simulink model "Alpha3"  (R2024a)
settings: Solver=FixedStepDiscrete  StartTime=0.0  StopTime=44100  RelTol=1e-3
PreLoadFcn:
  | t = linspace(0,256,4096)';
model workspace (MAT data in the model file):
  filter_nr_interpolations = Simulink.Parameter
  filter_nr_interpolations.Value = 4
  filter_nr_interpolations.Complexity = 'real'
  filter_nr_interpolations.Dimensions = [1 1]
  filter_nr_interpolations.Description = 'Number of interpolations applied by the low-pass filter'
  filter_nr_interpolations.DataType = 'uint8'
  max_hpf_cutoff_freq = Simulink.Parameter
  max_hpf_cutoff_freq.Value = 10000
  max_hpf_cutoff_freq.Complexity = 'real'
  max_hpf_cutoff_freq.Dimensions = [1 1]
  max_hpf_cutoff_freq.Description = 'Maximum cutoff frequency of the HPF
    | 
    | Defined by experiments.'
  max_hpf_cutoff_freq.DataType = 'uint16'
  max_resonance = Simulink.Parameter
  max_resonance.Value = 1.8
  max_resonance.Complexity = 'real'
  max_resonance.Dimensions = [1 1]
  max_resonance.DataType = 'auto'
  sampling_freq = Simulink.Parameter
  sampling_freq.Value = 44100
  sampling_freq.Complexity = 'real'
  sampling_freq.Dimensions = [1 1]
  sampling_freq.Description = 'Sampling frequency
    | 
    | Defines the tick period of the system.'
  sampling_freq.DataType = 'uint32'
  vmax = Simulink.Parameter
  vmax.Value = 1
  vmax.Complexity = 'real'
  vmax.Dimensions = [1 1]
  vmax.Description = 'Maximum sample value'
  vmax.DataType = 'auto'
  vmin = Simulink.Parameter
  vmin.Value = -1
  vmin.Complexity = 'real'
  vmin.Dimensions = [1 1]
  vmin.Description = 'Minimum sample value'
  vmin.DataType = 'auto'
  xtones = Simulink.Parameter
  xtones.Value = 252
  xtones.Complexity = 'real'
  xtones.Dimensions = [1 1]
  xtones.Description = 'Number of "x" tones in an octave
    | 
    | By default, an octave is 12 semi-tones.
    | To detune a frequency more finely, we divide an octave in a number of xtones, which should be a multiple of 12: x xtones is 12 semi-tones.
    | '
  xtones.DataType = 'int16'
libraries: dspsrcs4 x1
settings Model: NumberOfSteps=15  Creator=dfurodet  LastModifiedBy=dfurodet
settings DataIOCC: ExternalInput=[t]
settings OptimizationCC: DefaultParameterBehavior=Inlined  EnhancedBackFolding=on  PassReuseOutputArgsAs=Individual arguments  ZeroExternalMemoryAtStartup=off  ZeroInternalMemoryAtStartup=off  OptimizeBlockOrder=speed  DifferentSizesBufferReuse=on  OptimizationCustomize=off  EfficientTunableParamExpr=on
settings DebuggingCC: ParameterTunabilityLossMsg=error
settings SFSimCC: MATLABDynamicMemAlloc=off
settings RTWCC: Description=Embedded Coder  SystemTargetFile=ert.tlc  TemplateMakefile=ert_default_tmf  GPUComputeCapability=3.5
settings CodeAppCC: ForceParamTrailComments=on  IgnoreCustomStorageClasses=off  OperatorAnnotations=on  SimulinkDataObjDesc=on  SFDataObjDesc=on  InsertBlockDesc=on
settings ERTTargetCC: TargetLangStandard=C99 (ISO)  GenerateSampleERTMain=on  InlinedParameterPlacement=NonHierarchical  ERTCustomFileTemplate=example_file_process.tlc
settings ConfigComp: DVTestSuiteOptimization=Auto  DVDetectOutOfBounds=on  DVModelReferenceHarness=on  DVHarnessSource=Signal Editor

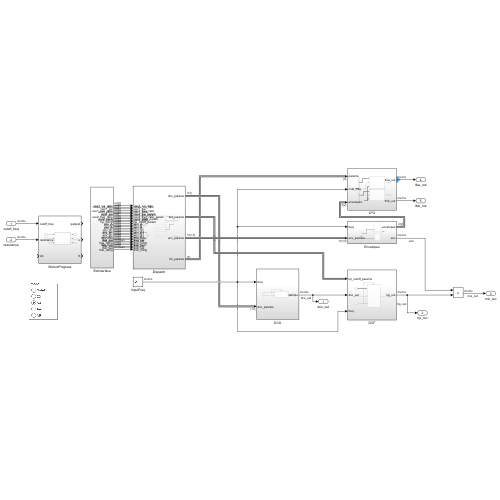
[thumbnail: Simulink's stored preview of the top-level diagram]
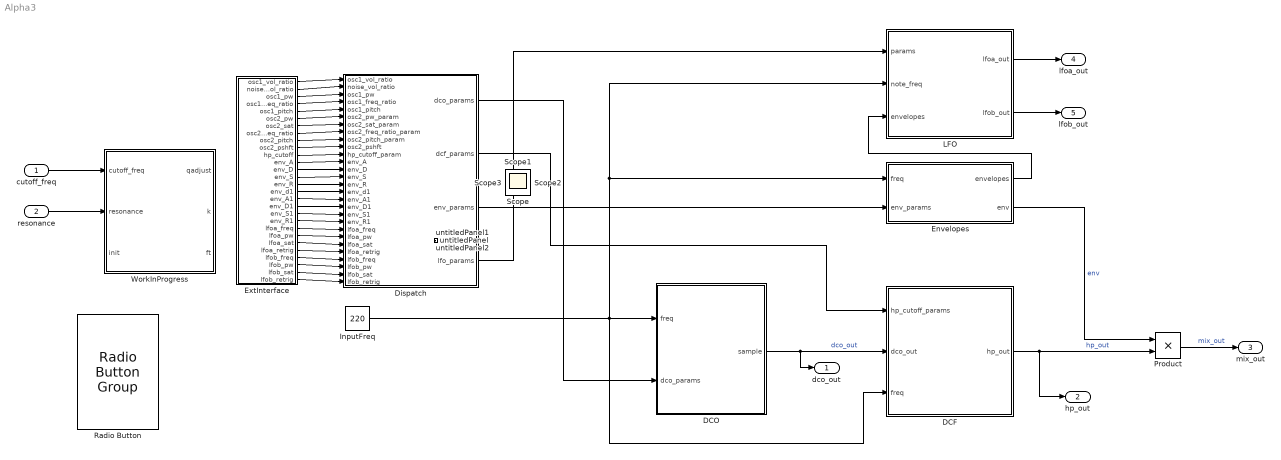
== system Alpha3 ==
  cutoff_freq : Inport
  resonance : Inport  Port=2
  DCF : Subsystem
  DCO : Subsystem
  Dispatch : Subsystem
  Envelopes : Subsystem
  ExtInterface : Subsystem
  InputFreq : Constant  Value=220
  LFO : Subsystem
  Product : Product
  Radio Button : RadioButtonGroup  LabelPosition=Hide  SelectedLabel=A3  ButtonGroupName=Mode
      settings: Values={{'NoteOff', 'C3', 'A3', 'A4', 'A5'}, [0 261.626 220 440 880]}
  WorkInProgress : Subsystem
  untitledPanel : Subsystem  Tag=HiddenForWebPanel  IsWebBlockPanel=on
  untitledPanel1 : Subsystem  Tag=HiddenForWebPanel  IsWebBlockPanel=on
  untitledPanel2 : Subsystem  Tag=HiddenForWebPanel  IsWebBlockPanel=on
  dco_out : Outport
  hp_out : Outport  Port=2
  mix_out : Outport  Port=3
  lfoa_out : Outport  Port=4
  lfob_out : Outport  Port=5
  Scope{,1..3} (4 alike) : Scope
  wires:
  DCO/1(sample) -> dco_out/1, DCF/2(dco_out)  "dco_out"
  ExtInterface/7(osc2_sat) -> Dispatch/7(osc2_sat_param)
  Dispatch/1(dco_params) -> DCO/2(dco_params)
  cutoff_freq/1 -> WorkInProgress/1(cutoff_freq)
  resonance/1 -> WorkInProgress/2(resonance)
  ExtInterface/11(hp_cutoff) -> Dispatch/11(hp_cutoff_param)
  Dispatch/2(dcf_params) -> DCF/1(hp_cutoff_params)
  DCF/1(hp_out) -> hp_out/1, Product/2  "hp_out"
  ExtInterface/1(osc1_vol_ratio) -> Dispatch/1(osc1_vol_ratio)
  ExtInterface/8(osc2_freq_ratio) -> Dispatch/8(osc2_freq_ratio_param)
  ExtInterface/6(osc2_pw) -> Dispatch/6(osc2_pw_param)
  ExtInterface/9(osc2_pitch) -> Dispatch/9(osc2_pitch_param)
  ExtInterface/10(osc2_pshft) -> Dispatch/10(osc2_pshft)
  ExtInterface/3(osc1_pw) -> Dispatch/3(osc1_pw)
  ExtInterface/4(osc1_freq_ratio) -> Dispatch/4(osc1_freq_ratio)
  ExtInterface/5(osc1_pitch) -> Dispatch/5(osc1_pitch)
  ExtInterface/2(noise_vol_ratio) -> Dispatch/2(noise_vol_ratio)
  InputFreq/1 -> DCO/1(freq), DCF/3(freq), LFO/2(note_freq), Envelopes/1(freq)
  Envelopes/2(env) -> Product/1  "env"
  Dispatch/3(env_params) -> Envelopes/2(env_params)
  ExtInterface/12(env_A) -> Dispatch/12(env_A)
  ExtInterface/13(env_D) -> Dispatch/13(env_D)
  ExtInterface/14(env_S) -> Dispatch/14(env_S)
  ExtInterface/15(env_R) -> Dispatch/15(env_R)
  ExtInterface/16(env_d1) -> Dispatch/16(env_d1)
  ExtInterface/17(env_A1) -> Dispatch/17(env_A1)
  ExtInterface/18(env_D1) -> Dispatch/18(env_D1)
  ExtInterface/19(env_S1) -> Dispatch/19(env_S1)
  ExtInterface/20(env_R1) -> Dispatch/20(env_R1)
  Product/1 -> mix_out/1  "mix_out"
  Dispatch/4(lfo_params) -> LFO/1(params)
  LFO/1(lfoa_out) -> lfoa_out/1
  LFO/2(lfob_out) -> lfob_out/1
  ExtInterface/21(lfoa_freq) -> Dispatch/21(lfoa_freq)
  ExtInterface/22(lfoa_pw) -> Dispatch/22(lfoa_pw)
  ExtInterface/23(lfoa_sat) -> Dispatch/23(lfoa_sat)
  ExtInterface/25(lfob_freq) -> Dispatch/25(lfob_freq)
  ExtInterface/26(lfob_pw) -> Dispatch/26(lfob_pw)
  ExtInterface/27(lfob_sat) -> Dispatch/27(lfob_sat)
  ExtInterface/24(lfoa_retrig) -> Dispatch/24(lfoa_retrig)
  ExtInterface/28(lfob_retrig) -> Dispatch/28(lfob_retrig)
  Envelopes/1(envelopes) -> LFO/3(envelopes)

== system Alpha3/DCF ==
  hp_cutoff_params : Inport
  dco_out : Inport  Port=2
  freq : Inport  Port=3
  Enabled Subsystem : Subsystem  TreatAsAtomicUnit=on
  hp_out : Outport
  wires:
  hp_cutoff_params/1 -> Enabled Subsystem/1(hp_cutoff_params)
  dco_out/1 -> Enabled Subsystem/2(sample)
  freq/1 -> Enabled Subsystem/3(freq), Enabled Subsystem/Enable
  Enabled Subsystem/1(hp_out) -> hp_out/1

== system Alpha3/DCO ==
  freq : Inport
  dco_params : Inport  Port=2
  Generate Sample : Subsystem  TreatAsAtomicUnit=on
  sample : Outport
  wires:
  freq/1 -> Generate Sample/Enable, Generate Sample/1(freq)
  dco_params/1 -> Generate Sample/2(dco_params)
  Generate Sample/1(sample) -> sample/1

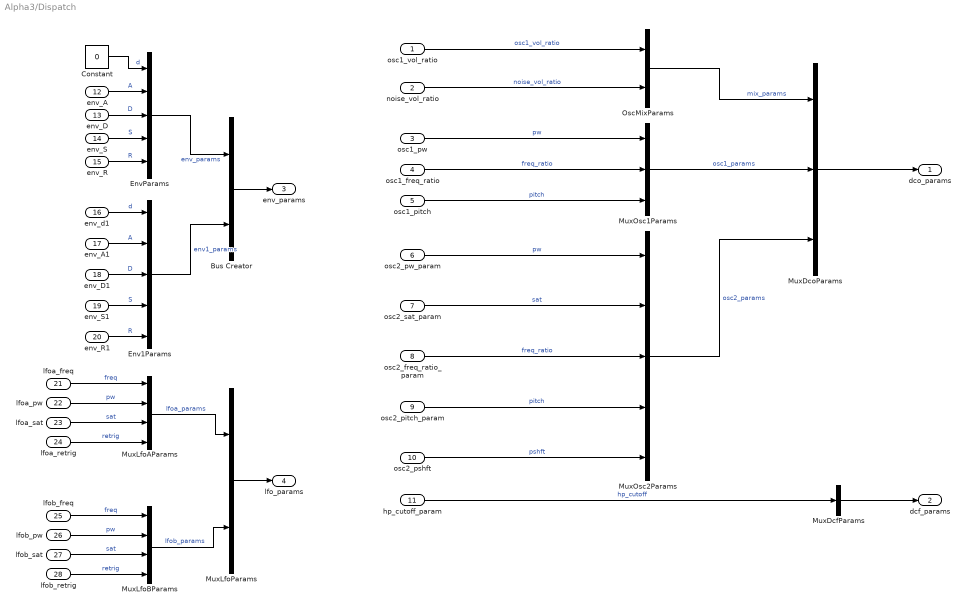
== system Alpha3/Dispatch ==
  osc1_vol_ratio : Inport
  noise_vol_ratio : Inport  Port=2
  osc1_pw : Inport  Port=3
  osc1_freq_ratio : Inport  Port=4
  osc1_pitch : Inport  Port=5
  osc2_pw_param : Inport  Port=6
  osc2_sat_param : Inport  Port=7
  osc2_freq_ratio_param : Inport  Port=8
  osc2_pitch_param : Inport  Port=9
  osc2_pshft : Inport  Port=10
  hp_cutoff_param : Inport  Port=11
  env_A : Inport  Port=12
  env_D : Inport  Port=13
  env_S : Inport  Port=14
  env_R : Inport  Port=15
  env_d1 : Inport  Port=16
  env_A1 : Inport  Port=17
  env_D1 : Inport  Port=18
  env_S1 : Inport  Port=19
  env_R1 : Inport  Port=20
  lfoa_freq : Inport  Port=21
  lfoa_pw : Inport  Port=22
  lfoa_sat : Inport  Port=23
  lfoa_retrig : Inport  Port=24
  lfob_freq : Inport  Port=25
  lfob_pw : Inport  Port=26
  lfob_sat : Inport  Port=27
  lfob_retrig : Inport  Port=28
  Bus Creator : BusCreator  Inputs=2
  Constant : Constant  Value=0  OutDataTypeStr=uint8
  Env1Params : BusCreator  Inputs=5
  EnvParams : BusCreator  Inputs=5
  MuxDcfParams : BusCreator  Inputs=1
  MuxDcoParams : BusCreator  Inputs=3
  MuxLfoAParams : BusCreator  Inputs=4
  MuxLfoBParams : BusCreator  Inputs=4
  MuxLfoParams : BusCreator  Inputs=2
  MuxOsc1Params : BusCreator  Inputs=3
  MuxOsc2Params : BusCreator  Inputs=5
  OscMixParams : BusCreator  Inputs=2
  dco_params : Outport
  dcf_params : Outport  Port=2
  env_params : Outport  Port=3
  lfo_params : Outport  Port=4
  wires:
  osc2_sat_param/1 -> MuxOsc2Params/2  "sat"
  MuxDcoParams/1 -> dco_params/1
  osc2_freq_ratio_param/1 -> MuxOsc2Params/3  "freq_ratio"
  MuxOsc2Params/1 -> MuxDcoParams/3  "osc2_params"
  osc2_pw_param/1 -> MuxOsc2Params/1  "pw"
  osc2_pitch_param/1 -> MuxOsc2Params/4  "pitch"
  osc2_pshft/1 -> MuxOsc2Params/5  "pshft"
  osc1_pw/1 -> MuxOsc1Params/1  "pw"
  MuxOsc1Params/1 -> MuxDcoParams/2  "osc1_params"
  osc1_freq_ratio/1 -> MuxOsc1Params/2  "freq_ratio"
  osc1_pitch/1 -> MuxOsc1Params/3  "pitch"
  noise_vol_ratio/1 -> OscMixParams/2  "noise_vol_ratio"
  osc1_vol_ratio/1 -> OscMixParams/1  "osc1_vol_ratio"
  OscMixParams/1 -> MuxDcoParams/1  "mix_params"
  MuxDcfParams/1 -> dcf_params/1
  hp_cutoff_param/1 -> MuxDcfParams/1  "hp_cutoff"
  env_A/1 -> EnvParams/2  "A"
  env_D/1 -> EnvParams/3  "D"
  env_S/1 -> EnvParams/4  "S"
  env_R/1 -> EnvParams/5  "R"
  env_R1/1 -> Env1Params/5  "R"
  env_D1/1 -> Env1Params/3  "D"
  env_S1/1 -> Env1Params/4  "S"
  env_A1/1 -> Env1Params/2  "A"
  env_d1/1 -> Env1Params/1  "d"
  EnvParams/1 -> Bus Creator/1  "env_params"
  Env1Params/1 -> Bus Creator/2  "env1_params"
  Bus Creator/1 -> env_params/1
  Constant/1 -> EnvParams/1  "d"
  lfoa_freq/1 -> MuxLfoAParams/1  "freq"
  lfoa_pw/1 -> MuxLfoAParams/2  "pw"
  lfoa_sat/1 -> MuxLfoAParams/3  "sat"
  lfob_freq/1 -> MuxLfoBParams/1  "freq"
  lfob_pw/1 -> MuxLfoBParams/2  "pw"
  lfob_sat/1 -> MuxLfoBParams/3  "sat"
  MuxLfoAParams/1 -> MuxLfoParams/1  "lfoa_params"
  MuxLfoBParams/1 -> MuxLfoParams/2  "lfob_params"
  MuxLfoParams/1 -> lfo_params/1
  lfoa_retrig/1 -> MuxLfoAParams/4  "retrig"
  lfob_retrig/1 -> MuxLfoBParams/4  "retrig"

== system Alpha3/Envelopes ==
  freq : Inport
  env_params : Inport  Port=2
  Bus Creator : BusCreator  Inputs=2
  Bus Selector : BusSelector  OutputSignals=env_params,env1_params
  Envelope : Subsystem  ReferencedSubsystem=Envelope
  Envelope1 : Subsystem  ReferencedSubsystem=Envelope
  envelopes : Outport
  env : Outport  Port=2
  wires:
  Envelope/1 -> Bus Creator/1, env/1  "env"
  freq/1 -> Envelope1/1, Envelope/1
  env_params/1 -> Bus Selector/1
  Bus Selector/1 -> Envelope/2  "<env_params>"
  Bus Selector/2 -> Envelope1/2  "<env1_params>"
  Envelope1/1 -> Bus Creator/2  "env1"
  Bus Creator/1 -> envelopes/1

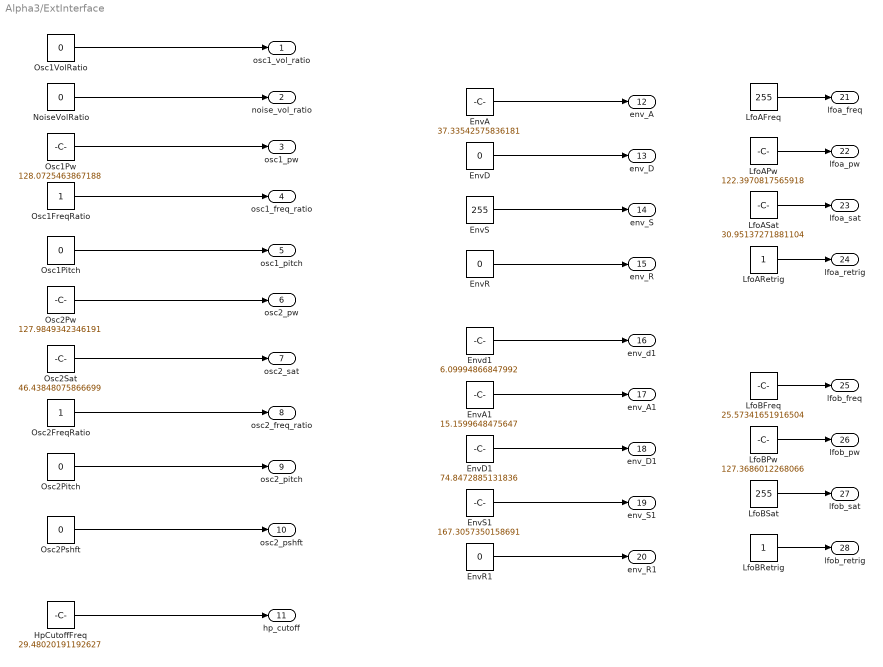
== system Alpha3/ExtInterface ==
  EnvA : Constant  Value=37.33542575836181  OutDataTypeStr=uint8
  EnvA1 : Constant  Value=15.1599648475647  OutDataTypeStr=uint8
  EnvD : Constant  Value=0  OutDataTypeStr=uint8
  EnvD1 : Constant  Value=74.8472885131836  OutDataTypeStr=uint8
  EnvR : Constant  Value=0  OutDataTypeStr=uint8
  EnvR1 : Constant  Value=0  OutDataTypeStr=uint8
  EnvS : Constant  Value=255  OutDataTypeStr=uint8
  EnvS1 : Constant  Value=167.3057350158691  OutDataTypeStr=uint8
  Envd1 : Constant  Value=6.09994866847992  OutDataTypeStr=uint8
  HpCutoffFreq : Constant  Value=29.48020191192627  OutMin=0  OutMax=255  OutDataTypeStr=uint8
  LfoAFreq : Constant  Value=255  OutDataTypeStr=uint8
  LfoAPw : Constant  Value=122.3970817565918  OutDataTypeStr=uint8
  LfoARetrig : Constant  OutDataTypeStr=boolean
  LfoASat : Constant  Value=30.95137271881104  OutDataTypeStr=uint8
  LfoBFreq : Constant  Value=25.57341651916504  OutDataTypeStr=uint8
  LfoBPw : Constant  Value=127.3686012268066  OutDataTypeStr=uint8
  LfoBRetrig : Constant  OutDataTypeStr=boolean
  LfoBSat : Constant  Value=255  OutDataTypeStr=uint8
  NoiseVolRatio : Constant  Value=0  OutDataTypeStr=uint8
  Osc1FreqRatio : Constant  OutDataTypeStr=half
  Osc1Pitch : Constant  Value=0  OutDataTypeStr=uint8
  Osc1Pw : Constant  Value=128.0725463867188  OutDataTypeStr=uint8
  Osc1VolRatio : Constant  Value=0  OutDataTypeStr=uint8
  Osc2FreqRatio : Constant  OutDataTypeStr=half
  Osc2Pitch : Constant  Value=0  OutDataTypeStr=uint8
  Osc2Pshft : Constant  Value=0  OutDataTypeStr=uint8
  Osc2Pw : Constant  Value=127.9849342346191  OutDataTypeStr=uint8
  Osc2Sat : Constant  Value=46.43848075866699  OutMin=0  OutMax=255  OutDataTypeStr=uint8
  osc1_vol_ratio : Outport
  noise_vol_ratio : Outport  Port=2
  osc1_pw : Outport  Port=3
  osc1_freq_ratio : Outport  Port=4
  osc1_pitch : Outport  Port=5
  osc2_pw : Outport  Port=6
  osc2_sat : Outport  Port=7
  osc2_freq_ratio : Outport  Port=8
  osc2_pitch : Outport  Port=9
  osc2_pshft : Outport  Port=10
  hp_cutoff : Outport  Port=11
  env_A : Outport  Port=12
  env_D : Outport  Port=13
  env_S : Outport  Port=14
  env_R : Outport  Port=15
  env_d1 : Outport  Port=16
  env_A1 : Outport  Port=17
  env_D1 : Outport  Port=18
  env_S1 : Outport  Port=19
  env_R1 : Outport  Port=20
  lfoa_freq : Outport  Port=21
  lfoa_pw : Outport  Port=22
  lfoa_sat : Outport  Port=23
  lfoa_retrig : Outport  Port=24
  lfob_freq : Outport  Port=25
  lfob_pw : Outport  Port=26
  lfob_sat : Outport  Port=27
  lfob_retrig : Outport  Port=28
  wires:
  Osc2Sat/1 -> osc2_sat/1
  HpCutoffFreq/1 -> hp_cutoff/1
  Osc1VolRatio/1 -> osc1_vol_ratio/1
  Osc2FreqRatio/1 -> osc2_freq_ratio/1
  Osc2Pw/1 -> osc2_pw/1
  Osc2Pitch/1 -> osc2_pitch/1
  Osc2Pshft/1 -> osc2_pshft/1
  Osc1Pw/1 -> osc1_pw/1
  Osc1Pitch/1 -> osc1_pitch/1
  Osc1FreqRatio/1 -> osc1_freq_ratio/1
  NoiseVolRatio/1 -> noise_vol_ratio/1
  EnvA/1 -> env_A/1
  EnvD/1 -> env_D/1
  EnvS/1 -> env_S/1
  EnvR/1 -> env_R/1
  EnvA1/1 -> env_A1/1
  EnvD1/1 -> env_D1/1
  Envd1/1 -> env_d1/1
  EnvS1/1 -> env_S1/1
  EnvR1/1 -> env_R1/1
  LfoAFreq/1 -> lfoa_freq/1
  LfoAPw/1 -> lfoa_pw/1
  LfoASat/1 -> lfoa_sat/1
  LfoBPw/1 -> lfob_pw/1
  LfoBSat/1 -> lfob_sat/1
  LfoBFreq/1 -> lfob_freq/1
  LfoARetrig/1 -> lfoa_retrig/1
  LfoBRetrig/1 -> lfob_retrig/1

== system Alpha3/LFO ==
  params : Inport
  note_freq : Inport  Port=2
  envelopes : Inport  Port=3
  Bus Selector : BusSelector  OutputSignals=lfoa_params,lfob_params
  LFO_A : Subsystem  ReferencedSubsystem=GenericLFO
  LFO_B : Subsystem  ReferencedSubsystem=GenericLFO
  lfoa_out : Outport
  lfob_out : Outport  Port=2
  wires:
  LFO_B/1 -> lfob_out/1
  params/1 -> Bus Selector/1
  Bus Selector/1 -> LFO_A/1  "<lfoa_params>"
  Bus Selector/2 -> LFO_B/1  "<lfob_params>"
  LFO_A/1 -> lfoa_out/1
  note_freq/1 -> LFO_B/2, LFO_A/2
  envelopes/1 -> LFO_B/3, LFO_A/3

== system Alpha3/WorkInProgress ==
  cutoff_freq : Inport
  resonance : Inport  Port=2
  init : Inport  Port=3
  LadderFilter : Subsystem
  qadjust : Outport
  k : Outport  Port=2
  ft : Outport  Port=3
  wires:
  resonance/1 -> LadderFilter/2(resonance)
  LadderFilter/1(qadjust) -> qadjust/1
  LadderFilter/2(k) -> k/1
  cutoff_freq/1 -> LadderFilter/1(cutoff_freq)
  init/1 -> LadderFilter/3(init)
  LadderFilter/3(ft) -> ft/1

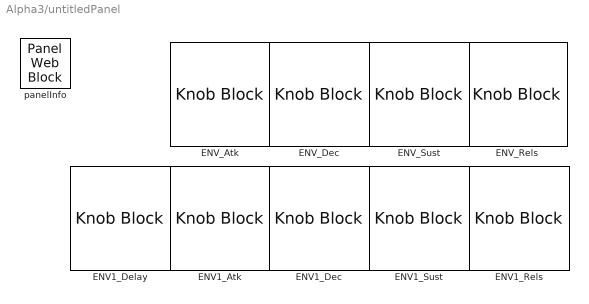
== system Alpha3/untitledPanel ==
  ENV1_Atk : KnobBlock  Tag=HiddenForWebPanel  PanelInfo="{\"height\":104,\"left\":165,\"panelId\":\"panelId-6f64585f-a0c9-4340-a288-a4a9f62721f3\",\"top\":143,\"type\":\"panelChild\",\"version\":\"2019b\",\"width\":100,\"zIndex\":1500010}"  LabelPosition=Hide  ScaleMax=255  TickInterval=32
  ENV1_Dec : KnobBlock  Tag=HiddenForWebPanel  PanelInfo="{\"height\":104,\"left\":264,\"panelId\":\"panelId-6f64585f-a0c9-4340-a288-a4a9f62721f3\",\"top\":143,\"type\":\"panelChild\",\"version\":\"2019b\",\"width\":100,\"zIndex\":1500012}"  LabelPosition=Hide  ScaleMax=255  TickInterval=32
  ENV1_Delay : KnobBlock  Tag=HiddenForWebPanel  PanelInfo="{\"height\":104,\"left\":65,\"panelId\":\"panelId-6f64585f-a0c9-4340-a288-a4a9f62721f3\",\"top\":143,\"type\":\"panelChild\",\"version\":\"2019b\",\"width\":100,\"zIndex\":1500018}"  LabelPosition=Hide  ScaleMax=255  TickInterval=32
  ENV1_Rels : KnobBlock  Tag=HiddenForWebPanel  PanelInfo="{\"height\":104,\"left\":464,\"panelId\":\"panelId-6f64585f-a0c9-4340-a288-a4a9f62721f3\",\"top\":143,\"type\":\"panelChild\",\"version\":\"2019b\",\"width\":100,\"zIndex\":1500016}"  LabelPosition=Hide  ScaleMax=255  TickInterval=32
  ENV1_Sust : KnobBlock  Tag=HiddenForWebPanel  PanelInfo="{\"height\":104,\"left\":364,\"panelId\":\"panelId-6f64585f-a0c9-4340-a288-a4a9f62721f3\",\"top\":143,\"type\":\"panelChild\",\"version\":\"2019b\",\"width\":100,\"zIndex\":1500014}"  LabelPosition=Hide  ScaleMax=255  TickInterval=32
  ENV_Atk : KnobBlock  Tag=HiddenForWebPanel  PanelInfo="{\"height\":104,\"left\":165,\"panelId\":\"panelId-6f64585f-a0c9-4340-a288-a4a9f62721f3\",\"top\":19,\"type\":\"panelChild\",\"version\":\"2019b\",\"width\":100,\"zIndex\":1500002}"  LabelPosition=Hide  ScaleMax=255  TickInterval=32
  ENV_Dec : KnobBlock  Tag=HiddenForWebPanel  PanelInfo="{\"height\":104,\"left\":264,\"panelId\":\"panelId-6f64585f-a0c9-4340-a288-a4a9f62721f3\",\"top\":19,\"type\":\"panelChild\",\"version\":\"2019b\",\"width\":100,\"zIndex\":1500004}"  LabelPosition=Hide  ScaleMax=255  TickInterval=32
  ENV_Rels : KnobBlock  Tag=HiddenForWebPanel  PanelInfo="{\"height\":104,\"left\":462,\"panelId\":\"panelId-6f64585f-a0c9-4340-a288-a4a9f62721f3\",\"top\":19,\"type\":\"panelChild\",\"version\":\"2019b\",\"width\":100,\"zIndex\":1500008}"  LabelPosition=Hide  ScaleMax=255  TickInterval=32
  ENV_Sust : KnobBlock  Tag=HiddenForWebPanel  PanelInfo="{\"height\":104,\"left\":364,\"panelId\":\"panelId-6f64585f-a0c9-4340-a288-a4a9f62721f3\",\"top\":19,\"type\":\"panelChild\",\"version\":\"2019b\",\"width\":100,\"zIndex\":1500006}"  LabelPosition=Hide  ScaleMax=255  TickInterval=32
  panelInfo : PanelWebBlock  Tag=HiddenForWebPanel  PanelInfo="{\"compacted\":true,\"height\":459,\"isActiveTab\":true,\"labels\":{\"label2040935304\":{\"deleted\":false,\"left\":293,\"settings\":{\"backgroundColor\":\"rgba(0, 0, 0, 0)\",\"bold\":true,\"font\":\"Arial\",\"fontColor\":\"black\",\"fontSize\":0.9,\"italicized\":false,\"underlined\":false},\"text\":\"Decay\",\"top\":123},\"label2545823007\":{\"deleted\":false,\"left\":93,\"settings\":{\"backgroundColor\":\"rgba(0, 0, 0, 0)\",\"bold\":true,\"font\":\"Arial\",\"fontColor\":\"black\",\"fontSize\":0.9,\"italicized\":false,\"underlined\":false},\"text\":\"Delay\",\"top\":248},\"label4541142813\":{\"deleted\":false,\"left\":388,\"settings\":{\"backgroundColor\":\"rgba(0, 0, 0, 0)\",\"bold\":true,\"font\":\"Arial\",\"fontColor\":\"black\",\"fontSize\":0.9,\"italicized\":false,\"underlined\":false},\"text\":\"Sustain\",\"top\":124},\"label4884836141\":{\"deleted\":false,\"left\":23,\"settings\":{\"backgroundColor\":\"rgba(0, 0, 0, 0)\",\"bold\":true,\"font\":\"Arial\",\"fontColor\":\"black\",\"fontSize\":0.9,\"italicized\":false,\"underlined\":false},\"text\":\"ENV1\",\"top\":146},\"label5439540327\":{\"deleted\":false,\"left\":490,\"settings\":{\"backgroundColor\":\"rgba(0, 0, 0, 0)\",\"bold\":true,\"font\":\"Arial\",\"fontColor\":\"black\",\"fontSize\":0.9,\"italicized\":false,\"underlined\":false},\"text\":\"Release\",\"top\":249},\"label5591963709\":{\"deleted\":false,\"left\":286,\"settings\":{\"backgroundColor\":\"rgba(0, 0, 0, 0)\",\"bold\":true,\"font\":\"Arial\",\"fontColor\":\"black\",\"fontSize\":0.9,\"italicized\":false,\"underlined\":false},\"text\":\"Decay\",\"top\":249},\"label8134870689\":{\"deleted\":false,\"left\":191,\"settings\":{\"backgroundColor\":\"rgba(0, 0, 0, 0)\",\"bold\":true,\"font\":\"Arial\",\"fontColor\":\"black\",\"fontSize\":0.9,\"italicized\":false,\"underlined\":false},\"text\":\"Attack\",\"top\":123},\"label8661865290\":{\"deleted\":false,\"left\":479,\"settings\":{\"backgroundColor\":\"rgba(0, 0, 0, 0)\",\"bold\":true,\"font\":\"Arial\",\"fontColor\":\"black\",\"fontSize\":0.9,\"italicized\":false,\"underlined\":false},\"text\":\"Release\",\"top\":124},\"label8818408462\":{\"deleted\":false,\"left\":128,\"settings\":{\"backgroundColor\":\"rgba(0, 0, 0, 0)\",\"bold\":true,\"font\":\"Arial\",\"fontColor\":\"black\",\"fontSize\":0.9,\"italicized\":false,\"underlined\":false},\"text\":\"ENV\",\"top\":21},\"label9023925417\":{\"deleted\":false,\"left\":190,\"settings\":{\"backgroundColor\":\"rgba(0, 0, 0, 0)\",\"bold\":true,\"font\":\"Arial\",\"fontColor\":\"black\",\"fontSize\":0.9,\"italicized\":false,\"underlined\":false},\"text\":\"Attack\",\"top\":248},\"label9886902808\":{\"deleted\":false,\"left\":383,\"settings\":{\"backgroundColor\":\"rgba(0, 0, 0, 0)\",\"bold\":true,\"font\":\"Arial\",\"fontColor\":\"black\",\"fontSize\":0.9,\"italicized\":false,\"underlined\":false},\"text\":\"Sustain\",\"top\":250}},\"left\":94,\"name\":\"Panel1\",\"panelId\":\"panelId-6f64585f-a0c9-4340-a288-a4a9f62721f3\",\"tabIndex\":1,\"tabbedSetId\":\"tabbedSet1624543179\",\"top\":32,\"type\":\"panel\",\"version\":\"2019b\",\"visible\":true,\"width\":1236,\"zIndex\":1500008}"  PanelSnapshot=<binary blob, 45756 chars, not shown>

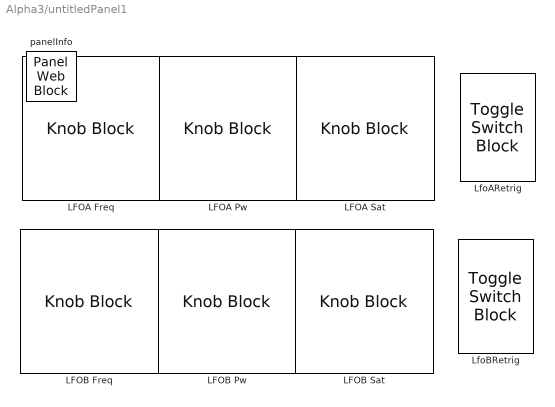
== system Alpha3/untitledPanel1 ==
  " LfoARetrig" : ToggleSwitchBlock  Tag=HiddenForWebPanel  PanelInfo="{\"height\":108,\"left\":446,\"panelId\":\"panelId-e79746d5-17de-49d0-a7d2-277f9aa122dc\",\"top\":42,\"type\":\"panelChild\",\"version\":\"2019b\",\"width\":75,\"zIndex\":1500014}"  LabelPosition=Hide
      settings: Values={{'FreeRunning', 'Retrig'}, [0 1]}
  " LfoBRetrig" : ToggleSwitchBlock  Tag=HiddenForWebPanel  PanelInfo="{\"height\":114,\"left\":447,\"panelId\":\"panelId-e79746d5-17de-49d0-a7d2-277f9aa122dc\",\"top\":203,\"type\":\"panelChild\",\"version\":\"2019b\",\"width\":75,\"zIndex\":1500016}"  LabelPosition=Hide
      settings: Values={{'FreeRunning', 'Retrig'}, [0 1]}
  LFOA Freq : KnobBlock  Tag=HiddenForWebPanel  PanelInfo="{\"height\":144,\"left\":11,\"panelId\":\"panelId-e79746d5-17de-49d0-a7d2-277f9aa122dc\",\"top\":20,\"type\":\"panelChild\",\"version\":\"2019b\",\"width\":138,\"zIndex\":1500002}"  LabelPosition=Hide  ScaleMax=255  TickInterval=32
  LFOA Pw : KnobBlock  Tag=HiddenForWebPanel  PanelInfo="{\"height\":144,\"left\":148,\"panelId\":\"panelId-e79746d5-17de-49d0-a7d2-277f9aa122dc\",\"top\":20,\"type\":\"panelChild\",\"version\":\"2019b\",\"width\":138,\"zIndex\":1500004}"  LabelPosition=Hide  ScaleMax=255  TickInterval=32
  LFOA Sat : KnobBlock  Tag=HiddenForWebPanel  PanelInfo="{\"height\":144,\"left\":285,\"panelId\":\"panelId-e79746d5-17de-49d0-a7d2-277f9aa122dc\",\"top\":20,\"type\":\"panelChild\",\"version\":\"2019b\",\"width\":138,\"zIndex\":1500006}"  LabelPosition=Hide  ScaleMax=255  TickInterval=32
  LFOB Freq : KnobBlock  Tag=HiddenForWebPanel  PanelInfo="{\"height\":144,\"left\":9,\"panelId\":\"panelId-e79746d5-17de-49d0-a7d2-277f9aa122dc\",\"top\":193,\"type\":\"panelChild\",\"version\":\"2019b\",\"width\":138,\"zIndex\":1500008}"  LabelPosition=Hide  ScaleMax=255  TickInterval=32
  LFOB Pw : KnobBlock  Tag=HiddenForWebPanel  PanelInfo="{\"height\":144,\"left\":147,\"panelId\":\"panelId-e79746d5-17de-49d0-a7d2-277f9aa122dc\",\"top\":193,\"type\":\"panelChild\",\"version\":\"2019b\",\"width\":138,\"zIndex\":1500010}"  LabelPosition=Hide  ScaleMax=255  TickInterval=32
  LFOB Sat : KnobBlock  Tag=HiddenForWebPanel  PanelInfo="{\"height\":144,\"left\":284,\"panelId\":\"panelId-e79746d5-17de-49d0-a7d2-277f9aa122dc\",\"top\":193,\"type\":\"panelChild\",\"version\":\"2019b\",\"width\":138,\"zIndex\":1500012}"  LabelPosition=Hide  ScaleMax=255  TickInterval=32
  panelInfo : PanelWebBlock  Tag=HiddenForWebPanel  PanelInfo="{\"compacted\":true,\"height\":538,\"isActiveTab\":false,\"labels\":{\"label4500295810\":{\"deleted\":false,\"left\":205,\"settings\":{\"backgroundColor\":\"rgba(0, 0, 0, 0)\",\"bold\":true,\"font\":\"Arial\",\"fontColor\":\"black\",\"fontSize\":0.9,\"italicized\":false,\"underlined\":false},\"text\":\"PW\",\"top\":337},\"label4841523118\":{\"deleted\":false,\"left\":340,\"settings\":{\"backgroundColor\":\"rgba(0, 0, 0, 0)\",\"bold\":true,\"font\":\"Arial\",\"fontColor\":\"black\",\"fontSize\":0.9,\"italicized\":false,\"underlined\":false},\"text\":\"SAT\",\"top\":336},\"label5017496792\":{\"deleted\":false,\"left\":207,\"settings\":{\"backgroundColor\":\"rgba(0, 0, 0, 0)\",\"bold\":true,\"font\":\"Arial\",\"fontColor\":\"black\",\"fontSize\":0.9,\"italicized\":false,\"underlined\":false},\"text\":\"PW\",\"top\":162},\"label6715147697\":{\"deleted\":false,\"left\":69,\"settings\":{\"backgroundColor\":\"rgba(0, 0, 0, 0)\",\"bold\":true,\"font\":\"Arial\",\"fontColor\":\"black\",\"fontSize\":0.9,\"italicized\":false,\"underlined\":false},\"text\":\"F\",\"top\":338},\"label7936683388\":{\"deleted\":false,\"left\":338,\"settings\":{\"backgroundColor\":\"rgba(0, 0, 0, 0)\",\"bold\":true,\"font\":\"Arial\",\"fontColor\":\"black\",\"fontSize\":0.9,\"italicized\":false,\"underlined\":false},\"text\":\"SAT\",\"top\":162},\"label8607232746\":{\"deleted\":false,\"left\":64,\"settings\":{\"backgroundColor\":\"rgba(0, 0, 0, 0)\",\"bold\":true,\"font\":\"Arial\",\"fontColor\":\"black\",\"fontSize\":0.9,\"italicized\":false,\"underlined\":false},\"text\":\"F\",\"top\":162}},\"left\":94,\"name\":\"Panel2\",\"panelId\":\"panelId-e79746d5-17de-49d0-a7d2-277f9aa122dc\",\"tabIndex\":2,\"tabbedSetId\":\"tabbedSet1624543179\",\"top\":32,\"type\":\"panel\",\"version\":\"2019b\",\"visible\":false,\"width\":1448,\"zIndex\":1500010}"  PanelSnapshot=<binary blob, 65524 chars, not shown>

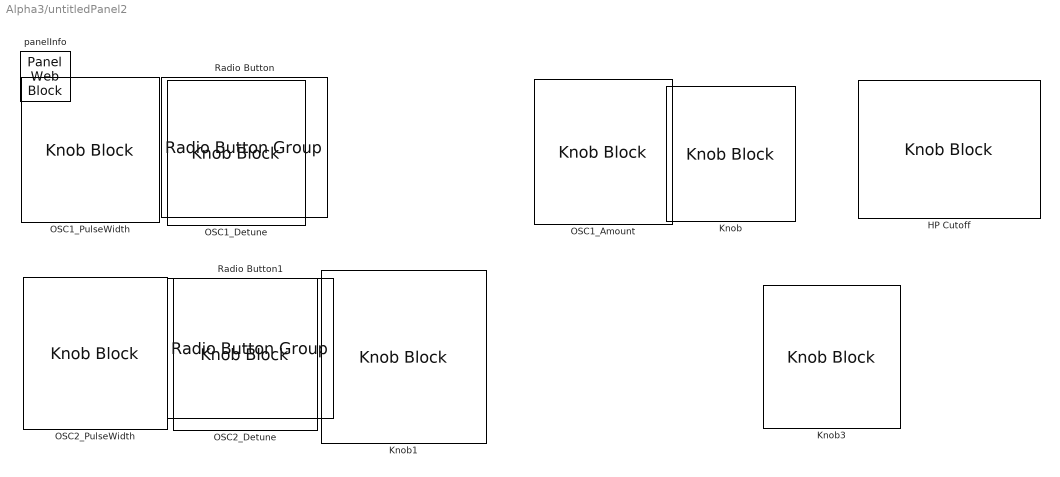
== system Alpha3/untitledPanel2 ==
  HP Cutoff : KnobBlock  Tag=HiddenForWebPanel  PanelInfo="{\"height\":138,\"left\":984,\"panelId\":\"panelId-d5c5c6ba-ae60-4cc1-a29a-bd08d6775c16\",\"top\":256,\"type\":\"panelChild\",\"version\":\"2019b\",\"width\":182,\"zIndex\":1500024}"  LabelPosition=Hide  ScaleMax=255  TickInterval=32
  Knob : KnobBlock  Tag=HiddenForWebPanel  PanelInfo="{\"height\":135,\"left\":661,\"panelId\":\"panelId-d5c5c6ba-ae60-4cc1-a29a-bd08d6775c16\",\"top\":50,\"type\":\"panelChild\",\"version\":\"2019b\",\"width\":129,\"zIndex\":1500026}"  ScaleMax=255
  Knob1 : KnobBlock  Tag=HiddenForWebPanel  PanelInfo="{\"height\":151,\"left\":474,\"panelId\":\"panelId-d5c5c6ba-ae60-4cc1-a29a-bd08d6775c16\",\"top\":245,\"type\":\"panelChild\",\"version\":\"2019b\",\"width\":142,\"zIndex\":1500014}"  LabelPosition=Hide  ScaleMax=255  TickInterval=32
  Knob3 : KnobBlock  Tag=HiddenForWebPanel  PanelInfo="{\"height\":143,\"left\":624,\"panelId\":\"panelId-d5c5c6ba-ae60-4cc1-a29a-bd08d6775c16\",\"top\":248,\"type\":\"panelChild\",\"version\":\"2019b\",\"width\":137,\"zIndex\":1500022}"  LabelPosition=Hide  ScaleMax=255  TickInterval=32
  OSC1_Amount : KnobBlock  Tag=HiddenForWebPanel  PanelInfo="{\"height\":145,\"left\":465,\"panelId\":\"panelId-d5c5c6ba-ae60-4cc1-a29a-bd08d6775c16\",\"top\":41,\"type\":\"panelChild\",\"version\":\"2019b\",\"width\":138,\"zIndex\":1500006}"  LabelPosition=Hide  ScaleMax=255  TickInterval=64
  OSC1_Detune : KnobBlock  Tag=HiddenForWebPanel  PanelInfo="{\"height\":145,\"left\":325,\"panelId\":\"panelId-d5c5c6ba-ae60-4cc1-a29a-bd08d6775c16\",\"top\":40,\"type\":\"panelChild\",\"version\":\"2019b\",\"width\":138,\"zIndex\":1500004}"  LabelPosition=Hide  ScaleMax=252  TickInterval=21
  OSC1_PulseWidth : KnobBlock  Tag=HiddenForWebPanel  PanelInfo="{\"height\":145,\"left\":16,\"panelId\":\"panelId-d5c5c6ba-ae60-4cc1-a29a-bd08d6775c16\",\"top\":41,\"type\":\"panelChild\",\"version\":\"2019b\",\"width\":138,\"zIndex\":1500002}"  LabelPosition=Hide  ScaleMax=255  TickInterval=32
  OSC2_Detune : KnobBlock  Tag=HiddenForWebPanel  PanelInfo="{\"height\":152,\"left\":329,\"panelId\":\"panelId-d5c5c6ba-ae60-4cc1-a29a-bd08d6775c16\",\"top\":244,\"type\":\"panelChild\",\"version\":\"2019b\",\"width\":144,\"zIndex\":1500012}"  LabelPosition=Hide  ScaleMax=252  TickInterval=21
  OSC2_PulseWidth : KnobBlock  Tag=HiddenForWebPanel  PanelInfo="{\"height\":152,\"left\":18,\"panelId\":\"panelId-d5c5c6ba-ae60-4cc1-a29a-bd08d6775c16\",\"top\":241,\"type\":\"panelChild\",\"version\":\"2019b\",\"width\":144,\"zIndex\":1500010}"  LabelPosition=Hide  ScaleMax=255  TickInterval=32
  Radio Button : RadioButtonGroup  Tag=HiddenForWebPanel  PanelInfo="{\"height\":140,\"left\":156,\"panelId\":\"panelId-d5c5c6ba-ae60-4cc1-a29a-bd08d6775c16\",\"top\":42,\"type\":\"panelChild\",\"version\":\"2019b\",\"width\":166,\"zIndex\":1500018}"  LabelPosition=Hide  SelectedLabel=Oct  ButtonGroupName=OSC1 Detune
      settings: Values={{'Oct', 'Oct-1', 'Oct-2', 'Oct+1'}, [1 2 4 0.5]}
  Radio Button1 : RadioButtonGroup  Tag=HiddenForWebPanel  PanelInfo="{\"height\":140,\"left\":162,\"panelId\":\"panelId-d5c5c6ba-ae60-4cc1-a29a-bd08d6775c16\",\"top\":242,\"type\":\"panelChild\",\"version\":\"2019b\",\"width\":166,\"zIndex\":1500020}"  LabelPosition=Hide  SelectedLabel=Oct  ButtonGroupName=OSC2 Detune
      settings: Values={{'Oct', 'Oct-1', 'Oct-2', 'Oct+1'}, [1 2 4 0.5]}
  panelInfo : PanelWebBlock  Tag=HiddenForWebPanel  PanelInfo="{\"compacted\":true,\"height\":459,\"isActiveTab\":false,\"labels\":{\"label0559829798\":{\"deleted\":false,\"left\":704,\"settings\":{\"backgroundColor\":\"rgba(0, 0, 0, 0)\",\"bold\":true,\"font\":\"Arial\",\"fontColor\":\"black\",\"fontSize\":0.9,\"italicized\":false,\"underlined\":false},\"text\":\"Noise\",\"top\":189},\"label0753907431\":{\"deleted\":false,\"id\":\"label0753907431\",\"left\":300,\"settings\":{\"backgroundColor\":\"rgba(0, 0, 0, 0)\",\"bold\":true,\"font\":\"Arial\",\"fontColor\":\"black\",\"fontSize\":0.9,\"italicized\":false,\"underlined\":false},\"text\":\"DETUNE\",\"top\":436},\"label0799912635\":{\"deleted\":false,\"id\":\"label0799912635\",\"left\":471,\"settings\":{\"backgroundColor\":\"rgba(0, 0, 0, 0)\",\"bold\":true,\"font\":\"Arial\",\"fontColor\":\"black\",\"fontSize\":0.9,\"italicized\":false,\"underlined\":false},\"text\":\"VOLUME RATIO\",\"top\":190},\"label2544205989\":{\"deleted\":false,\"id\":\"label2544205989\",\"left\":301,\"settings\":{\"backgroundColor\":\"rgba(0, 0, 0, 0)\",\"bold\":true,\"font\":\"Arial\",\"fontColor\":\"black\",\"fontSize\":0.9,\"italicized\":false,\"underlined\":false},\"text\":\"DETUNE\",\"top\":190},\"label2742837468\":{\"deleted\":false,\"id\":\"label2742837468\",\"left\":393,\"settings\":{\"backgroundColor\":\"rgba(0, 0, 0, 0)\",\"bold\":true,\"font\":\"Arial\",\"fontColor\":\"black\",\"fontSize\":0.9,\"italicized\":false,\"underlined\":false},\"text\":\"PITCH\",\"top\":403},\"label2828133017\":{\"deleted\":false,\"id\":\"label2828133017\",\"left\":493,\"settings\":{\"backgroundColor\":\"rgba(0, 0, 0, 0)\",\"bold\":true,\"font\":\"Arial\",\"fontColor\":\"black\",\"fontSize\":0.9,\"italicized\":false,\"underlined\":false},\"text\":\"PHASE SHIFT\",\"top\":404},\"label4888191476\":{\"deleted\":false,\"id\":\"label4888191476\",\"left\":21,\"settings\":{\"backgroundColor\":\"rgba(0, 0, 0, 0)\",\"bold\":true,\"font\":\"Arial\",\"fontColor\":\"#aa0000\",\"fontSize\":0.9,\"italicized\":false,\"underlined\":false},\"text\":\"OSC2\",\"top\":219},\"label6556143853\":{\"deleted\":false,\"id\":\"label6556143853\",\"left\":78,\"settings\":{\"backgroundColor\":\"rgba(0, 0, 0, 0)\",\"bold\":true,\"font\":\"Arial\",\"fontColor\":\"black\",\"fontSize\":0.9,\"italicized\":false,\"underlined\":false},\"text\":\"PW\",\"top\":189},\"label6918991668\":{\"deleted\":false,\"id\":\"label6918991668\",\"left\":656,\"settings\":{\"backgroundColor\":\"rgba(0, 0, 0, 0)\",\"bold\":true,\"font\":\"Arial\",\"fontColor\":\"black\",\"fontSize\":0.9,\"italicized\":false,\"underlined\":false},\"text\":\"Saturation\",\"top\":400},\"label7711699721\":{\"deleted\":false,\"id\":\"label7711699721\",\"left\":80,\"settings\":{\"backgroundColor\":\"rgba(0, 0, 0, 0)\",\"bold\":true,\"font\":\"Arial\",\"fontColor\":\"black\",\"fontSize\":0.9,\"italicized\":false,\"underlined\":false},\"text\":\"PW\",\"top\":399},\"label8621024817\":{\"deleted\":false,\"id\":\"label8621024817\",\"left\":1036,\"settings\":{\"backgroundColor\":\"rgba(0, 0, 0, 0)\",\"bold\":true,\"font\":\"Arial\",\"fontColor\":\"black\",\"fontSize\":0.9,\"italicized\":false,\"underlined\":false},\"text\":\"HP Cutoff\",\"top\":409},\"label8790180575\":{\"deleted\":false,\"id\":\"label8790180575\",\"left\":21,\"settings\":{\"backgroundColor\":\"rgba(0, 0, 0, 0)\",\"bold\":true,\"font\":\"Arial\",\"fontColor\":\"#aa0000\",\"fontSize\":0.9,\"italicized\":false,\"underlined\":false},\"text\":\"OSC1\",\"top\":20}},\"left\":94,\"name\":\"Panel\",\"panelId\":\"panelId-d5c5c6ba-ae60-4cc1-a29a-bd08d6775c16\",\"tabIndex\":0,\"tabbedSetId\":\"tabbedSet1624543179\",\"top\":32,\"type\":\"panel\",\"version\":\"2019b\",\"visible\":false,\"width\":1236,\"zIndex\":1500006}"  PanelSnapshot=<binary blob, 164136 chars, not shown>

== system Alpha3/DCF/Enabled Subsystem ==
  hp_cutoff_params : Inport
  sample : Inport  Port=2
  freq : Inport  Port=3
  Enable : EnablePort
  Filters : Subsystem
  hp_out : Outport
  wires:
  hp_cutoff_params/1 -> Filters/1(hp_cutoff_params)
  sample/1 -> Filters/2(dco_out)
  freq/1 -> Filters/3(freq)
  Filters/1(hp_out) -> hp_out/1

== system Alpha3/DCO/Generate Sample ==
  freq : Inport
  dco_params : Inport  Port=2
  Enable : EnablePort
  Oscillators : Subsystem
  sample : Outport
  wires:
  dco_params/1 -> Oscillators/2(dco_params)
  Oscillators/1(sample) -> sample/1
  freq/1 -> Oscillators/1(freq)

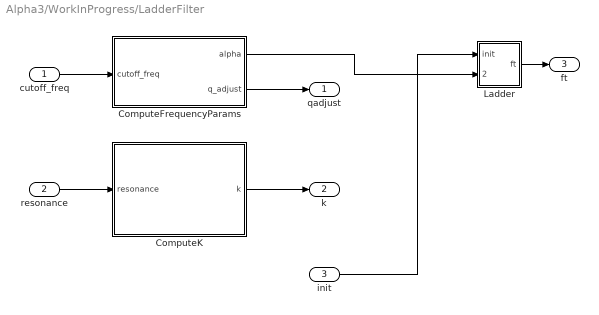
== system Alpha3/WorkInProgress/LadderFilter ==
  cutoff_freq : Inport
  resonance : Inport  Port=2
  init : Inport  Port=3
  ComputeFrequencyParams : Subsystem
  ComputeK : Subsystem
  Ladder : Subsystem
  qadjust : Outport
  k : Outport  Port=2
  ft : Outport  Port=3
  wires:
  cutoff_freq/1 -> ComputeFrequencyParams/1(cutoff_freq)
  ComputeFrequencyParams/2(q_adjust) -> qadjust/1
  ComputeK/1(k) -> k/1
  resonance/1 -> ComputeK/1(resonance)
  init/1 -> Ladder/1(init)
  Ladder/1(ft) -> ft/1
  ComputeFrequencyParams/1(alpha) -> Ladder/2(alpha)

== system Alpha3/DCF/Enabled Subsystem/Filters ==
  hp_cutoff_params : Inport
  dco_out : Inport  Port=2
  freq : Inport  Port=3
  Bus Selector : BusSelector  OutputSignals=hp_cutoff
  HPF : Subsystem  Description=|
      | Simple Butterworth filter of order 1 that implements an HPF
      | 
      | Minimum cutoff frequency is forced to 1 (which means no cutoff).
      | Maximum cutoff frequency is arbitrarily set to half of the sample rate, which already removes a lot of frequencies.
  hp_out : Outport
  wires:
  Bus Selector/1 -> HPF/1(hp_cutoff_freq)  "<hp_cutoff>"
  dco_out/1 -> HPF/2(sample)
  freq/1 -> HPF/3(freq)
  HPF/1(hpf_out) -> hp_out/1  "hp_out"
  hp_cutoff_params/1 -> Bus Selector/1

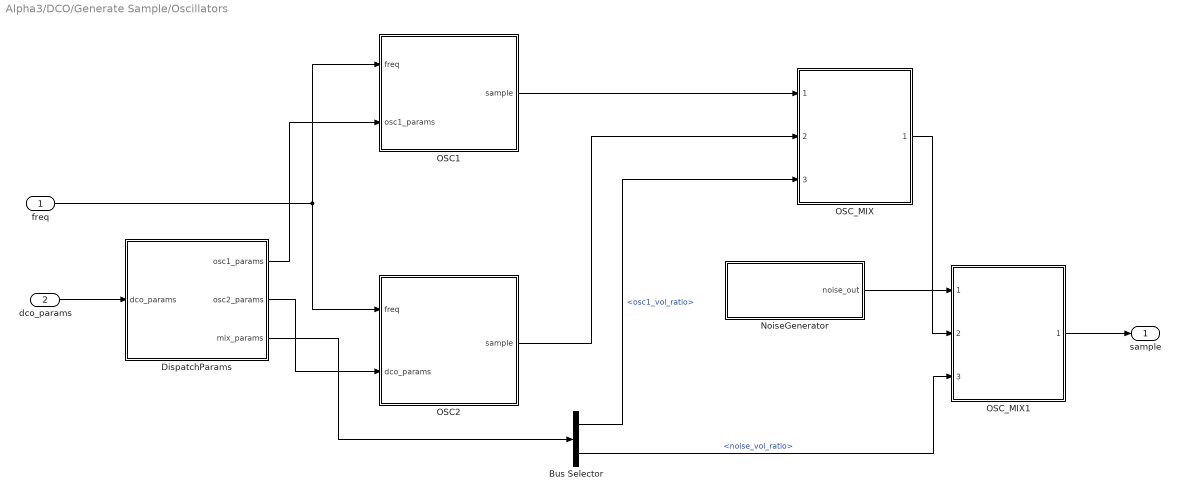
== system Alpha3/DCO/Generate Sample/Oscillators ==
  freq : Inport
  dco_params : Inport  Port=2
  Bus Selector : BusSelector  OutputSignals=osc1_vol_ratio,noise_vol_ratio
  DispatchParams : Subsystem
  NoiseGenerator : Subsystem
  OSC1 : Subsystem  mask{wave_len=256}
  OSC2 : Subsystem  mask{wave_len=2048}
  OSC_MIX : Subsystem  ReferencedSubsystem=MixSamples
  OSC_MIX1 : Subsystem  ReferencedSubsystem=MixSamples
  sample : Outport
  wires:
  OSC2/1(sample) -> OSC_MIX/2
  OSC1/1(sample) -> OSC_MIX/1
  freq/1 -> OSC1/1(freq), OSC2/1(freq)
  dco_params/1 -> DispatchParams/1(dco_params)
  DispatchParams/2(osc2_params) -> OSC2/2(dco_params)
  DispatchParams/1(osc1_params) -> OSC1/2(osc1_params)
  DispatchParams/3(mix_params) -> Bus Selector/1
  Bus Selector/1 -> OSC_MIX/3  "<osc1_vol_ratio>"
  OSC_MIX/1 -> OSC_MIX1/2
  Bus Selector/2 -> OSC_MIX1/3  "<noise_vol_ratio>"
  OSC_MIX1/1 -> sample/1
  NoiseGenerator/1(noise_out) -> OSC_MIX1/1

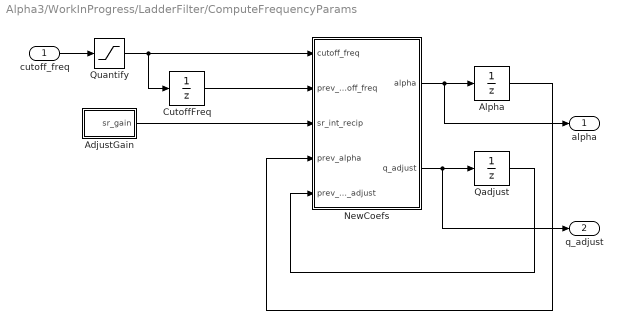
== system Alpha3/WorkInProgress/LadderFilter/ComputeFrequencyParams ==
  cutoff_freq : Inport
  AdjustGain : Subsystem
  Alpha : UnitDelay  SampleTime=-1  HasFrameUpgradeWarning=on
  CutoffFreq : UnitDelay  SampleTime=-1  HasFrameUpgradeWarning=on
  NewCoefs : MATLAB Function  TreatAsAtomicUnit=on
  Qadjust : UnitDelay  SampleTime=-1  HasFrameUpgradeWarning=on
  Quantify : Saturate  UpperLimit=0.425 * sampling_freq  LowerLimit=5
  alpha : Outport
  q_adjust : Outport  Port=2
  wires:
  cutoff_freq/1 -> Quantify/1
  Quantify/1 -> NewCoefs/1(cutoff_freq), CutoffFreq/1
  NewCoefs/2(q_adjust) -> q_adjust/1, Qadjust/1
  CutoffFreq/1 -> NewCoefs/2(prev_cutoff_freq)
  NewCoefs/1(alpha) -> alpha/1, Alpha/1
  Qadjust/1 -> NewCoefs/5(prev_q_adjust)
  Alpha/1 -> NewCoefs/4(prev_alpha)
  AdjustGain/1(sr_gain) -> NewCoefs/3(sr_int_recip)

== system Alpha3/WorkInProgress/LadderFilter/ComputeK ==
  resonance : Inport
  NewCoefs : MATLAB Function  TreatAsAtomicUnit=on
  Saturation : Saturate  UpperLimit=max_resonance  LowerLimit=0.0
  Unit Delay : UnitDelay  SampleTime=-1  HasFrameUpgradeWarning=on
  Unit Delay1 : UnitDelay  SampleTime=-1  HasFrameUpgradeWarning=on
  k : Outport
  wires:
  Unit Delay/1 -> NewCoefs/3(prev_k)
  NewCoefs/1(k) -> k/1, Unit Delay/1
  Unit Delay1/1 -> NewCoefs/2(prev_resonance)
  resonance/1 -> Saturation/1
  Saturation/1 -> Unit Delay1/1, NewCoefs/1(resonance)

== system Alpha3/WorkInProgress/LadderFilter/Ladder ==
  init : Inport
  alpha : Inport  Port=2
  Stage{1..4} (4 alike) : Subsystem  ReferencedSubsystem=LadderUnitLPF
  ft : Outport
  wires:
  Stage3/1 -> Stage4/1
  alpha/1 -> Stage4/2, Stage3/2, Stage2/2, Stage1/2
  init/1 -> Stage1/1
  Stage2/1 -> Stage3/1
  Stage4/1 -> ft/1
  Stage1/1 -> Stage2/1

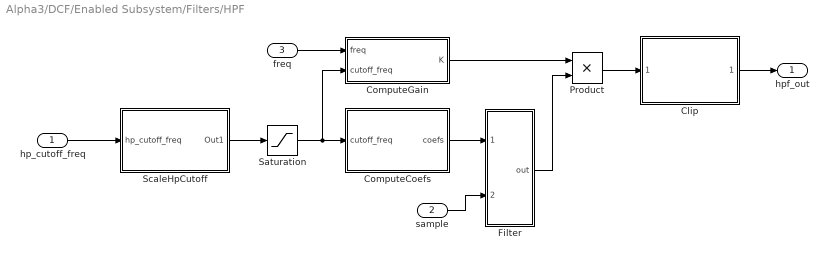
== system Alpha3/DCF/Enabled Subsystem/Filters/HPF ==
  hp_cutoff_freq : Inport
  sample : Inport  Port=2
  freq : Inport  Port=3
  Clip : Subsystem  ReferencedSubsystem=Clip
  ComputeCoefs : Subsystem
  ComputeGain : Subsystem
  Filter : Subsystem
  Product : Product
  Saturation : Saturate  UpperLimit=max_hpf_cutoff_freq  LowerLimit=1
  ScaleHpCutoff : Subsystem
  hpf_out : Outport
  wires:
  hp_cutoff_freq/1 -> ScaleHpCutoff/1(hp_cutoff_freq)
  freq/1 -> ComputeGain/1(freq)
  sample/1 -> Filter/2(sample)
  ScaleHpCutoff/1(Out1) -> Saturation/1
  Saturation/1 -> ComputeGain/2(cutoff_freq), ComputeCoefs/1(cutoff_freq)
  ComputeGain/1(K) -> Product/1
  ComputeCoefs/1(coefs) -> Filter/1(coefs)
  Filter/1(out) -> Product/2
  Product/1 -> Clip/1
  Clip/1 -> hpf_out/1

== system Alpha3/DCO/Generate Sample/Oscillators/DispatchParams ==
  dco_params : Inport
  Bus Selector : BusSelector  OutputSignals=osc1_params
  SelectMixParams : BusSelector  OutputSignals=mix_params
  SelectOsc2Params : BusSelector  OutputSignals=osc2_params
  osc1_params : Outport
  osc2_params : Outport  Port=2
  mix_params : Outport  Port=3
  wires:
  dco_params/1 -> Bus Selector/1, SelectOsc2Params/1, SelectMixParams/1
  SelectMixParams/1 -> mix_params/1  "<mix_params>"
  SelectOsc2Params/1 -> osc2_params/1  "<osc2_params>"
  Bus Selector/1 -> osc1_params/1  "<osc1_params>"

== system Alpha3/DCO/Generate Sample/Oscillators/NoiseGenerator ==
  " Dumb Extraction" : MATLAB Function  TreatAsAtomicUnit=on
  Colored Noise : dspsrcs4/Colored Noise  Color=blue  InverseFrequencyPower=1  BoundedOutput=on  NumChannels=1  OutputDataType=double  SamplesPerFrame=1  SampleTime=1  RandomStream=mt19937ar with seed  Seed=67  SimulateUsing=Code generation
  noise_out : Outport
  wires:
  " Dumb Extraction"/1(y) -> noise_out/1
  Colored Noise/1 -> " Dumb Extraction"/1(u)

== system Alpha3/DCO/Generate Sample/Oscillators/OSC1 ==
  freq : Inport
  osc1_params : Inport  Port=2
  OSC1_PROCESS : Subsystem
  sample : Outport
  wires:
  osc1_params/1 -> OSC1_PROCESS/1(osc1_params)
  freq/1 -> OSC1_PROCESS/2(freq)
  OSC1_PROCESS/1(sample) -> sample/1

== system Alpha3/DCO/Generate Sample/Oscillators/OSC2 ==
  freq : Inport
  dco_params : Inport  Port=2
  OSC2_PROCESS : Subsystem
  sample : Outport
  wires:
  freq/1 -> OSC2_PROCESS/1(freq)
  OSC2_PROCESS/1(sample) -> sample/1
  dco_params/1 -> OSC2_PROCESS/2(dco_params)

== system Alpha3/WorkInProgress/LadderFilter/ComputeFrequencyParams/AdjustGain ==
  Constant : Constant  Value=filter_nr_interpolations  OutDataTypeStr=uint8
  Constant1 : Constant
  Data Type Conversion : DataTypeConversion  OutDataTypeStr=double  SaturateOnIntegerOverflow=off  RndMeth=Floor
  Divide : Product  Inputs=*/
  Product : Product
  SamplingFreq : Constant  Value=sampling_freq
  sr_gain : Outport
  wires:
  Divide/1 -> sr_gain/1
  Data Type Conversion/1 -> Divide/2
  Constant/1 -> Product/2
  SamplingFreq/1 -> Product/1
  Constant1/1 -> Divide/1
  Product/1 -> Data Type Conversion/1

== system Alpha3/DCF/Enabled Subsystem/Filters/HPF/ComputeCoefs ==
  cutoff_freq : Inport
  Compute HPF Coefs : Subsystem  TreatAsAtomicUnit=on
  Equal : RelationalOperator  Operator=~=  RndMeth=Simplest  InputSameDT=off
  Unit Delay : UnitDelay  SampleTime=-1  HasFrameUpgradeWarning=on
  coefs : Outport
  wires:
  cutoff_freq/1 -> Equal/1, Compute HPF Coefs/1(cutoff_freq), Unit Delay/1
  Unit Delay/1 -> Equal/2
  Equal/1 -> Compute HPF Coefs/Trigger
  Compute HPF Coefs/1(hp_coefs) -> coefs/1

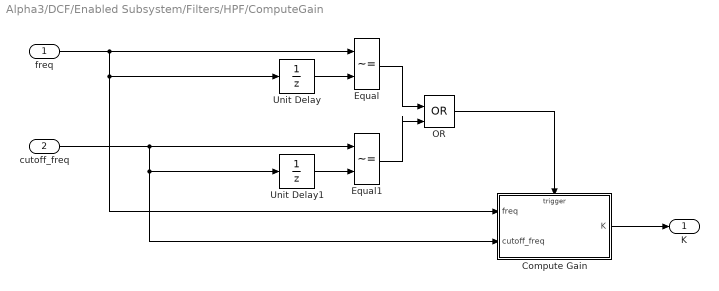
== system Alpha3/DCF/Enabled Subsystem/Filters/HPF/ComputeGain ==
  freq : Inport
  cutoff_freq : Inport  Port=2
  Compute Gain : Subsystem  TreatAsAtomicUnit=on
  Equal : RelationalOperator  Operator=~=  OutDataTypeStr=boolean  RndMeth=Simplest  InputSameDT=off
  Equal1 : RelationalOperator  Operator=~=  OutDataTypeStr=boolean  RndMeth=Simplest  InputSameDT=off
  OR : Logic  Operator=OR  IconShape=distinctive  AllPortsSameDT=off  OutDataTypeStr=boolean
  Unit Delay : UnitDelay  SampleTime=-1  HasFrameUpgradeWarning=on
  Unit Delay1 : UnitDelay  SampleTime=-1  HasFrameUpgradeWarning=on
  K : Outport
  wires:
  freq/1 -> Compute Gain/1(freq), Unit Delay/1, Equal/1
  cutoff_freq/1 -> Compute Gain/2(cutoff_freq), Unit Delay1/1, Equal1/1
  Unit Delay/1 -> Equal/2
  Unit Delay1/1 -> Equal1/2
  Equal/1 -> OR/1
  Equal1/1 -> OR/2
  OR/1 -> Compute Gain/Trigger
  Compute Gain/1(K) -> K/1

== system Alpha3/DCF/Enabled Subsystem/Filters/HPF/Filter ==
  coefs : Inport
  sample : Inport  Port=2
  Bus Selector : BusSelector  OutputSignals=A,D1,D2
  Hpf : MATLAB Function  TreatAsAtomicUnit=on
  Unit Delay : UnitDelay  SampleTime=-1  HasFrameUpgradeWarning=on
  Unit Delay1 : UnitDelay  SampleTime=-1  HasFrameUpgradeWarning=on
  out : Outport
  wires:
  Hpf/1(out) -> out/1
  sample/1 -> Hpf/6(sample)
  Hpf/2(w0_out) -> Unit Delay/1
  Unit Delay/1 -> Hpf/4(w1), Unit Delay1/1
  Unit Delay1/1 -> Hpf/5(w2)
  coefs/1 -> Bus Selector/1
  Bus Selector/1 -> Hpf/1(a)  "<A>"
  Bus Selector/2 -> Hpf/2(d1)  "<D1>"
  Bus Selector/3 -> Hpf/3(d2)  "<D2>"

== system Alpha3/DCF/Enabled Subsystem/Filters/HPF/ScaleHpCutoff ==
  hp_cutoff_freq : Inport
  Data Type Conversion : DataTypeConversion  OutDataTypeStr=uint32  SaturateOnIntegerOverflow=off  RndMeth=Floor
  Divide : Product  Inputs=*/
  MaxHpCutoff : Constant  Value=max_hpf_cutoff_freq
  MaxParamValue : Constant  Value="intmax(\"uint8\") + 1"  OutDataTypeStr=uint32
  Product : Product
  Out1 : Outport
  wires:
  Data Type Conversion/1 -> Product/1
  MaxParamValue/1 -> Divide/2
  Product/1 -> Divide/1
  MaxHpCutoff/1 -> Product/2
  Divide/1 -> Out1/1
  hp_cutoff_freq/1 -> Data Type Conversion/1

== system Alpha3/DCO/Generate Sample/Oscillators/OSC1/OSC1_PROCESS ==
  osc1_params : Inport
  freq : Inport  Port=2
  Bus Selector : BusSelector  OutputSignals=pw,freq_ratio,pitch
  OSC1_PW : Subsystem  ReferencedSubsystem=PWMOsc
  OSC1_SAMPLING : Subsystem
  sample : Outport
  wires:
  OSC1_PW/1 -> OSC1_SAMPLING/3(PW)
  OSC1_SAMPLING/1(sample) -> sample/1
  Bus Selector/3 -> OSC1_SAMPLING/4(pitch)  "<pitch>"
  freq/1 -> OSC1_SAMPLING/1(freq)
  Bus Selector/2 -> OSC1_SAMPLING/2(freq_ratio)  "<freq_ratio>"
  osc1_params/1 -> Bus Selector/1
  Bus Selector/1 -> OSC1_PW/1  "<pw>"

== system Alpha3/DCO/Generate Sample/Oscillators/OSC2/OSC2_PROCESS ==
  freq : Inport
  dco_params : Inport  Port=2
  DemuxParams : BusSelector  OutputSignals=pw,sat,freq_ratio,pitch,pshft
  OSC2_PW : Subsystem  ReferencedSubsystem=PWMOsc
  OSC2_SAMPLING : Subsystem
  sample : Outport
  wires:
  OSC2_PW/1 -> OSC2_SAMPLING/3(PW)
  OSC2_SAMPLING/1(sample) -> sample/1
  freq/1 -> OSC2_SAMPLING/1(freq)
  dco_params/1 -> DemuxParams/1
  DemuxParams/2 -> OSC2_SAMPLING/6(sat)  "<sat>"
  DemuxParams/3 -> OSC2_SAMPLING/2(freq_ratio)  "<freq_ratio>"
  DemuxParams/1 -> OSC2_PW/1  "<pw>"
  DemuxParams/4 -> OSC2_SAMPLING/4(pitch)  "<pitch>"
  DemuxParams/5 -> OSC2_SAMPLING/5(pshft)  "<pshft>"

== system Alpha3/DCF/Enabled Subsystem/Filters/HPF/ComputeCoefs/Compute HPF Coefs ==
  cutoff_freq : Inport
  Trigger : TriggerPort  VariantControl=(inherit)  InitialTriggerSignalState=zero
  Bus Creator : BusCreator  Inputs=3
  Constant : Constant  Value=sampling_freq
  HPOrder1Coefs : MATLAB Function  TreatAsAtomicUnit=on
  hp_coefs : Outport
  wires:
  Bus Creator/1 -> hp_coefs/1
  HPOrder1Coefs/3(D2) -> Bus Creator/3
  HPOrder1Coefs/1(A) -> Bus Creator/1
  cutoff_freq/1 -> HPOrder1Coefs/1(cutoff_freq)
  HPOrder1Coefs/2(D1) -> Bus Creator/2
  Constant/1 -> HPOrder1Coefs/2(sampling_freq)

== system Alpha3/DCF/Enabled Subsystem/Filters/HPF/ComputeGain/Compute Gain ==
  freq : Inport
  cutoff_freq : Inport  Port=2
  Trigger : TriggerPort  VariantControl=(inherit)  InitialTriggerSignalState=zero
  " ComputeGain" : MATLAB Function  TreatAsAtomicUnit=on
  K : Outport
  wires:
  freq/1 -> " ComputeGain"/1(fs)
  cutoff_freq/1 -> " ComputeGain"/2(fc)
  " ComputeGain"/1(K) -> K/1

== system Alpha3/DCO/Generate Sample/Oscillators/OSC1/OSC1_PROCESS/OSC1_SAMPLING ==
  freq : Inport
  freq_ratio : Inport  Port=2
  PW : Inport  Port=3
  pitch : Inport  Port=4
  Constant : Constant  Value=0
  FrequencyIn : Subsystem  ReferencedSubsystem=FrequencyIn
  SquareOsc : Subsystem
  sample : Outport
  wires:
  PW/1 -> SquareOsc/2(PW)
  Constant/1 -> FrequencyIn/4
  pitch/1 -> FrequencyIn/3
  freq_ratio/1 -> FrequencyIn/2
  freq/1 -> FrequencyIn/1
  FrequencyIn/1 -> SquareOsc/1(SampleId)
  SquareOsc/1(sample) -> sample/1

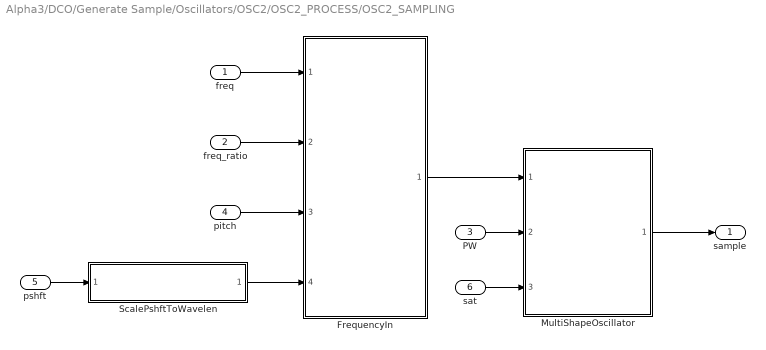
== system Alpha3/DCO/Generate Sample/Oscillators/OSC2/OSC2_PROCESS/OSC2_SAMPLING ==
  freq : Inport
  freq_ratio : Inport  Port=2
  PW : Inport  Port=3
  pitch : Inport  Port=4
  pshft : Inport  Port=5
  sat : Inport  Port=6
  FrequencyIn : Subsystem  ReferencedSubsystem=FrequencyIn
  MultiShapeOscillator : Subsystem  ReferencedSubsystem=MultiShapeOscillator
  ScalePshftToWavelen : Subsystem  ReferencedSubsystem=ScaleParamToWavelen
  sample : Outport
  wires:
  freq/1 -> FrequencyIn/1
  freq_ratio/1 -> FrequencyIn/2
  pshft/1 -> ScalePshftToWavelen/1
  ScalePshftToWavelen/1 -> FrequencyIn/4
  pitch/1 -> FrequencyIn/3
  FrequencyIn/1 -> MultiShapeOscillator/1
  PW/1 -> MultiShapeOscillator/2
  sat/1 -> MultiShapeOscillator/3
  MultiShapeOscillator/1 -> sample/1

== system Alpha3/DCO/Generate Sample/Oscillators/OSC1/OSC1_PROCESS/OSC1_SAMPLING/SquareOsc ==
  SampleId : Inport
  PW : Inport  Port=2
  Square : MATLAB Function  TreatAsAtomicUnit=on
  sample : Outport
  wires:
  PW/1 -> Square/2(pw)
  SampleId/1 -> Square/1(id)
  Square/1(sample) -> sample/1

== matlab function Alpha3/DCF/Enabled Subsystem/Filters/HPF/ComputeCoefs/Compute HPF Coefs/HPOrder1Coefs ==
  data: cutoff_freq input; A output; sampling_freq input; D1 output; D2 output
function [A, D1, D2] = hp_coeffs(cutoff_freq, sampling_freq)
a = tan(pi*(double(cutoff_freq) / 2) / double(sampling_freq));
a2 = a * a;
r = sin(pi / 4);
s = a2 + 2*a*r + 1;
A = 1/s;
D1 = 2 * (1 - a2) / s;
D2 = - (a2 - 2*a*r + 1) / s;

== matlab function Alpha3/WorkInProgress/LadderFilter/ComputeK/NewCoefs ==
  data: resonance input; k output; prev_resonance input; prev_k input
function k = compute_params(resonance, prev_resonance, prev_k)
if resonance == prev_resonance
    k = prev_k;
else
    k = 4.0 * resonance;
end

== matlab function Alpha3/DCF/Enabled Subsystem/Filters/HPF/ComputeGain/Compute Gain/ ComputeGain ==
  data: fs input; K output; fc input
function K = compute_gain(fs, fc)
r = double(fc)/fs;
h=sqrt(1/(1+r*r));
Gdb=-20*log10(h);
K=power(10,Gdb/20);

== matlab function Alpha3/DCO/Generate Sample/Oscillators/NoiseGenerator/ Dumb Extraction ==
  data: u input; y output
function y = fcn(u)
y = u(1);

== matlab function Alpha3/WorkInProgress/LadderFilter/ComputeFrequencyParams/NewCoefs ==
  data: cutoff_freq input; prev_cutoff_freq input; sr_int_recip input; alpha output; q_adjust output; prev_alpha input; prev_q_adjust input
function [alpha, q_adjust]= compute_coefs(cutoff_freq, prev_cutoff_freq, sr_int_recip, prev_alpha, prev_q_adjust)
if cutoff_freq == prev_cutoff_freq
    alpha = prev_alpha;
    q_adjust = prev_q_adjust;
else
    wc = cutoff_freq * 2.0 * pi * sr_int_recip;
    wc2 = wc * wc;
    alpha = 0.9892 * wc - 0.4324 * wc2 + 0.1381 * wc * wc2 - 0.0202 * wc2 * wc2;
    q_adjust = 1.006 + 0.0536 * wc - 0.095 * wc2 - 0.05 * wc2 * wc2;
end

== matlab function Alpha3/DCF/Enabled Subsystem/Filters/HPF/Filter/Hpf ==
  data: out output; a input; d1 input; d2 input; w0_out output; w1 input; w2 input; sample input
function [out, w0_out] = hpf(a, d1, d2, w1, w2, sample)
w0_out = d1 * w1 + d2 * w2 + sample;
out = a * (w0_out - 2 * w1 + w2);

== matlab function Alpha3/DCO/Generate Sample/Oscillators/OSC1/OSC1_PROCESS/OSC1_SAMPLING/SquareOsc/Square ==
  data: id input; sample output; pw input; wave_len parameter; vmin parameter; vmax parameter
function sample = square_signal(id, pw, wave_len, vmin, vmax)
if (pw == wave_len - 1) || (pw == 0)
    sample = 0;
elseif id < pw
    sample = vmin;
else
    sample = vmax;
end
